simulink model "AF_Sim_March_27"  (R2019b)
settings: Solver=VariableStepAuto  StartTime=0.0  StopTime=200  RelTol=1e-3
values from neighbouring files (symbols this model uses):
  u0 = [ 1.29  -0.1174  0  0]    [AF_Sim_Init.m]    (also in EOM.m = [1.29, -0.1174, 0, 0, -0.0153]; LiftDragMoment.m = [P Q R V beta alpha mu gamma chi zeta eta h]; testrun.m = [1.29, -0.1174, 0,  0, 64.828,     0,  -0.0153, 0,  0,  0,  )
  uin = [0, 0, 0, 0]    [AF_Sim_Init.m]    (also in LiftDragMoment.m = [d_th d_e d_r d_a]; testrun.m = zeros(1,16))
libraries: simulink x1
settings Model: Creator=hyeokjae  LastModifiedBy=chris
settings DebuggingCC: UnderSpecifiedDimensionMsg=warning
settings SFSimCC: CustomCodeUndefinedFunction=UseInterfaceOnly

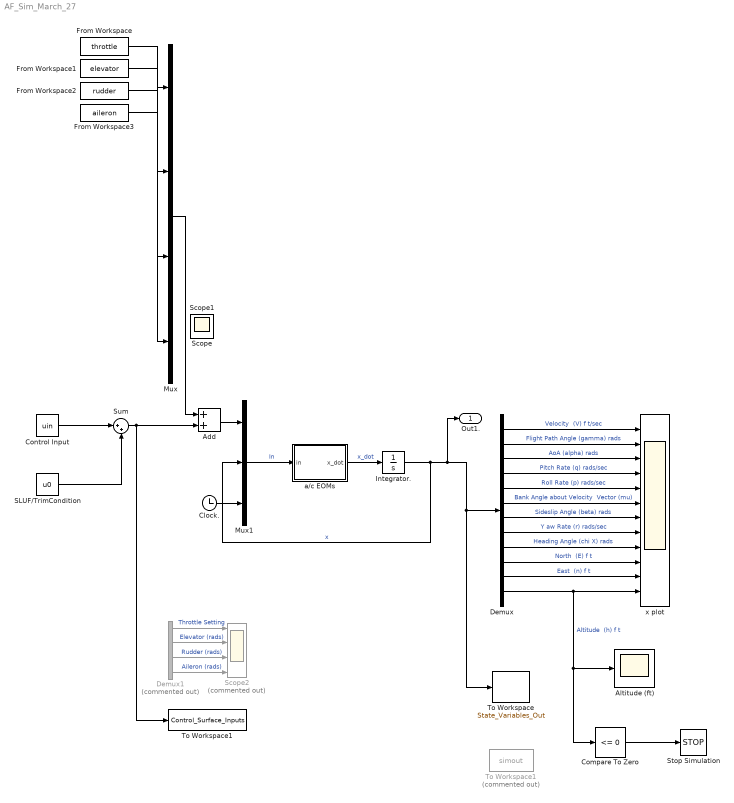
== system AF_Sim_March_27 ==
  Add : Sum
  Altitude (ft) : Scope
  Clock. : Clock
      settings: Decimation=100
  "Compare To Zero " : simulink/Logic and Bit Operations/Compare To Zero  relop=<=  OutDataTypeStr=boolean
  Control Input : Constant  Value=uin
  Demux : Demux  Outputs=12
  Demux1 : Demux  Commented=on
  From Workspace : FromWorkspace  VariableName=throttle  SampleTime=300
  From Workspace1 : FromWorkspace  VariableName=elevator  SampleTime=300
  From Workspace2 : FromWorkspace  VariableName=rudder  SampleTime=300
  From Workspace3 : FromWorkspace  VariableName=aileron  SampleTime=300
  Integrator. : Integrator
  Mux : Mux
  Mux1 : Mux  Inputs=3
  "SLUF/TrimCondition " : Constant  Value=u0
  Scope2 : Scope  Commented=on  NumInputPorts=4
  "Stop Simulation " : Stop
  Sum : Sum  Inputs=|++
  "To Workspace " : ToWorkspace  VariableName=State_Variables_Out  SampleTime=-1
      settings: Save2DSignal=2-D array (concatenate along first dimension)
  To Workspace1 : ToWorkspace  Commented=on  VariableName=simout  SaveFormat=Timeseries  SampleTime=-1
  "To Workspace1 " : ToWorkspace  VariableName=Control_Surface_Inputs  SampleTime=-1
      settings: Save2DSignal=2-D array (concatenate along first dimension)
  a/c EOMs : MATLAB Function  TreatAsAtomicUnit=on
  x plot : Scope  NumInputPorts=12
  Out1. : Outport  VectorParamsAs1DForOutWhenUnconnected=off
  Scope : Scope
  Scope1 : Scope
  wires:
  Control Input/1 -> Sum/1
  "SLUF/TrimCondition "/1 -> Sum/2
  Sum/1 -> "To Workspace1 "/1, Add/2
  Mux1/1 -> a/c EOMs/1(in)  "In"
  a/c EOMs/1(x_dot) -> Integrator./1  "x_dot"
  Integrator./1 -> Mux1/2, Out1./1, "To Workspace "/1, Demux/1  "x"
  Demux/1 -> x plot/1  "Velocity  (V) f t/sec"
  Demux/2 -> x plot/2  "Flight Path Angle (gamma) rads"
  Demux/3 -> x plot/3  "AoA (alpha) rads"
  Demux/4 -> x plot/4  "Pitch Rate (q) rads/sec"
  Demux/5 -> x plot/5  "Roll Rate (p) rads/sec"
  Demux/6 -> x plot/6  "Bank Angle about Velocity  Vector (mu)"
  Demux/7 -> x plot/7  "Sideslip Angle (beta) rads"
  Demux/8 -> x plot/8  "Y aw Rate (r) rads/sec"
  Demux/9 -> x plot/9  "Heading Angle (chi X) rads"
  Demux/10 -> x plot/10  "North  (E) f t"
  Demux/11 -> x plot/11  "East  (n) f t"
  Demux/12 -> "Compare To Zero "/1, Altitude (ft)/1, x plot/12  "Altitude  (h) f t"
  Clock./1 -> Mux1/3
  "Compare To Zero "/1 -> "Stop Simulation "/1
  Demux1/1 -> Scope2/1  "Throttle Setting"
  Demux1/2 -> Scope2/2  "Elevator (rads)"
  Demux1/3 -> Scope2/3  "Rudder (rads)"
  Demux1/4 -> Scope2/4  "Aileron (rads)"
  Add/1 -> Mux1/1
  Mux/1 -> Add/1
  From Workspace/1 -> Mux/1
  From Workspace3/1 -> Mux/4
  From Workspace2/1 -> Mux/3
  From Workspace1/1 -> Mux/2

== matlab function AF_Sim_March_27/a//c EOMs ==
  data: in input; x_dot output
function x_dot = fcn(in)

%AERE 531 Modified Sweep Angle Group
%This function takes inputs in the form of trim conditions (throttle, rudder, elevator...
%and aileron) and control input and outputs flight derivatives for use
%in the simulink model

%The equations used below are grouped together (17-25) and (26-33) as referrenced
%in "Development of Small Unmanned Aerial Vehicle Research Platform:
%Modeling and Simulating with Flight Test Validation"

%global manuever alpha_dot;
x_dot = zeros(12,1);

alpha_dot = 0;

%temporary input vector
%u0 = [1.29, -0.1174, 0,  0, 64.828,     0,  -0.0153, 0,  0,  0,     0, 0,   0,     0,    0, 1119, 100];
    % [T,     de,    dr, da, V,      gamma,  AoA,     q,  p, mu,  beta, r, chi, north, east,    h, clock-input]
   

   
%in = u0;


% PARSING INPUTS
%=============================================================
T   = in(1); %Thrust
de  = in(2); %Elevator deflection (down is +) {deg}
drt = in(3); %Rudder deflection {deg}
da  = in(4); %Aileron deflection {deg}

V       = in(5);  %Velocity {ft/s}
gamma   = in(6);  %Flight path angle {rad}
alpha   = in(7);  %Angle of attack {rad}
q       = in(8);  %Pitch Rate {rad/s}
p       = in(9);  %Roll Rate {rad/s}
mu      = in(10); %Bank Angle (About Velocity Vector) {rad}
beta    = in(11); %Sideslip Angle {rad}
r       = in(12); %Yaw Rate {rad/s}
chi     = in(13); %Heading angle {rads}
north   = in(14); %North Position {ft}
east    = in(15); %East Position {ft}
h       = in(16); %Altitude {ft}

tm = in(17);

% ATMOSPHERIC PROPERTIES
%=============================================================
rho = 0.0023081;    %Air Density (slugs per ft^3) -> do we want to make this a function of height?
g = 32.17;          %ft/s^2


% AIRCRAFT PROPERTIES
%==============================================================


m = 0.487669;       %Slugs - empty mass w/o fuel
Iyy = 1.5523;       %Inertia found with empty mass
Ixx = 1.948;        %Inertia
Izz = 1.9166;       %Inertia
Ixz = 0;            %Assumed zero due to symmetric aircraft

S = 10.56;          %Wing area - square feet
b = 9.16;           % Wing span - feet


CLow = 0.421;       %Wing coefficient of lift at 0deg AoA
CLaw = 4.59;        %Wing coefficient of lift per AoA
CDminw = 0.011;     %wing minimum coefficient of drag
ARw = (b^2)/S;      %Wing aspect ratio
e = 0.75;           %Span efficiency - ESTIMATION
Kw = 1/(pi*ARw*e);  %
Cmw = -0.005;       %Wing moment coefficient
cgw = -(5/12);      %Distance aero center is back from cg - 5 inches
c = (16/12);        %Root chord of wing (16") - feet
lambda = 0.72955;   %Taper ratio from S = (Cr*(1+lambda)*b)/2
CLat = 0.76;        %Vert tail coefficient of lift per AoA
CDmint = 0.002;     %vert tail minimum coeffcient of drag
Kt = 0.446;         %TO DO - MORE CALC?
it = deg2rad(2);    %Tail incidence 2 degrees to radians
Te = 0.422;         %Tail control surface effectiveness (??)
nt = 1;             %??
St = S;             %Horizontal tail area square feet = ref area (??)
cgt = 3.5;          %Distance tail aero center back from a/c cg

CLavt = 0.0969;     %Vertical tail coefficient of lift per AoA(??)
CDminvt = 0.001;    %vert tail min coefficient of drag (??)
Svt = S;            %Ref area of vertical tail = ref area (??)
Tr = 0.434;         %Name??
nvt = nt;           %same as hori tail (??)
cgvt = cgt;         %same as hori tail (??)

Cmaf = 0.114;       %fuselage moment coefficient
CDf = 0.005;        %Fuselage coefficient of drag

Cnda = -0.0128;     %per rad (??)
Clda = 0.244;       %per rad (??)


%Eqns 17-25
%Calculating necessary coefficients for use in Lift, Drag, and Moment
%equations
CLw=CLow+CLaw*alpha; %Coefficient of lift due to wing
CDw=CDminw+Kw*CLw^2; %Coefficient of drag due to wing
E=2*(CLow+CLaw*(alpha-alpha_dot*(cgt+cgw)/V))/(pi*ARw); %Not sure what to call this variable
alphat=alpha+it+Te*de+q*cgt/V-E; %angle of attack at horizontal tail
CLt=CLat*alphat; %Coefficient of lift due to horizonatl tail
CDt=CDmint+Kt*CLt^2; %Coefficient of drag due to horizontal tail
Cmf=Cmaf*alpha; %Moment coefficient due to fueselage 
CDvt=CDminvt; %Coefficient of drag due to vertical tail
Clp=-1/12*CLaw*(1+3*lambda)/(1+lambda); 

Clb=-.1; %rolling moment coefficient due to sideslip beta
Clr=.01;

%Eqns 26 - 33
%Forces and moments due to wing, horizontal and vertical tail, and
%fuselage:
qb=.5*rho*V^2; %q bar (dynamic pressure)
Lw=qb*S*CLw;   %lift due to wing
Dw=qb*S*CDw;   %drag due to wing
Mw=qb*S*c*Cmw; %pitching moment due to wing
Lt=nt*qb*St*CLt; %lift due to horizontal tail
Dt=nt*qb*St*CDt; %drag due to horizontal tai
Df=qb*S*CDf;    %drag due to fuselage
Mf=qb*S*c*Cmf;  %moment due to fuselage
Dvt=nt*qb*Svt*CDvt; %drag due to vertical tail

% Calculate Forces and Moments
% Total Lift
L=Lw+Lt*cos(E-q*cgt/V)-(Dt+Dvt)*sin(E-q*cgt/V);
% Total Drag
D=Dw+(Dt+Dvt)*cos(E-q*cgt/V)+Lt*sin(E-q*cgt/V)+Df;
% Total Side Force
Y=nvt*qb*Svt*CLavt*(-beta+Tr*drt+r*cgvt/V);
% Total Pitching Moment
Mc=Lw*cgw*cos(alpha)+Dw*cgw*sin(alpha)+Mw-Lt*cgt*cos(alpha-E+q*cgt/V)-(Dt+Dvt)*cgt*sin(alpha-E+q*cgt/V)+Mf;
% Total Yaw Moment
Nc=-qb*nvt*Svt*CLavt*(-beta+Tr*drt+r*cgvt/V)*cgvt+(-qb*S*b*Cnda*da);
% Total Roll Moment
Lc=qb*S*b^2/(2*V)*(Clp*p+2*V/b*Clb*beta+Clr*drt+Clda*da*2*V/b);




% -=-=-=-=-=- NONLINEAR 6-DOF EQUATION OF MOTION (EOMs) -=-=-=-=-=-=-=-=-
%
% These are the state derivative equations; the comment names the state,
% but the equation is for its derivative (rate)
%
% The equations are arranged by aircraft mode
%
% NOTE: These assume that Ixz=0, if not, then eq's need to be modified
% Longitudinal (phugoid and short period): V, gamma, q, alpha
% Phugoid: V, gamma
 % Velocity
 V_dot=1/m*(-D*cos(beta)+Y*sin(beta)+T*cos(beta)*cos(alpha))-...
 g*sin(gamma);
 % Flight Path Angle
 gamma_dot=1/(m*V)*(-D*sin(beta)*sin(mu)-Y*sin(mu)*cos(beta)...
 +L*cos(mu)+T*(cos(mu)*sin(alpha)+sin(mu)*sin(beta)*cos(alpha)))...
 -g/V*cos(gamma);
% Short Period: alpha, q
 % Angle of Attach
 alpha_dot=q-tan(beta)*(p*cos(alpha)+r*sin(alpha))-1/(m*V*cos(beta))...
 *(L+T*sin(alpha))+g*cos(gamma)*cos(mu)/(V*cos(beta));
 % Pitch Rate
 q_dot=Mc/Iyy+1/Iyy*(Izz*p*r-Ixx*r*p);
% Lateral (roll) - Directional (yaw): p, mu, beta, r
% Roll: p, mu
 % Roll Rate
 p_dot=Lc/Ixx+1/Ixx*(Iyy*r*q-Izz*q*r);

 % Bank Angle (about velocity vector)
 mu_dot=1/cos(beta)*(p*cos(alpha)+r*sin(alpha))+1/(m*V)*(D*sin(beta)...
 *cos(mu)*tan(gamma)+Y*tan(gamma)*cos(mu)*cos(beta)+L*(tan(beta)+...
 tan(gamma)*sin(mu))+T*(sin(alpha)*tan(gamma)*sin(mu)+sin(alpha)*...
 tan(beta)-cos(alpha)*tan(gamma)*cos(mu)*sin(beta)))-...
 g/V*cos(gamma)*cos(mu)*tan(beta);

% Dutch Roll: beta, r
 % Side Slip Angle
 beta_dot=-r*cos(alpha)+p*sin(alpha)+1/(m*V)*(D*sin(beta)+Y*cos...
 (beta)-T*sin(beta)*cos(alpha))+g/V*cos(gamma)*sin(mu);

 % Yaw Rate

 r_dot=Nc/Izz+1/Izz*(Ixx*p*q-Iyy*p*q);

% Heading Angle (from North)
 chi_dot=1/(m*V*cos(gamma))*(D*sin(beta)*cos(mu)+Y*cos(mu)*cos(beta)...
 +L*sin(mu)+T*(sin(mu)*sin(alpha)-cos(mu)*sin(beta)*cos(alpha)));

% Kinematic Equations
 % North Position
 n_dot=V*cos(gamma)*cos(chi);

 % East Position
 e_dot=V*cos(gamma)*sin(chi);

 % Altitude
 h_dot=V*sin(gamma);

% Pack derivatives into output vector x_dot
 x_dot(1) = V_dot;
 x_dot(2) = gamma_dot;
 x_dot(3) = alpha_dot;
 x_dot(4) = q_dot;
 x_dot(5) = p_dot;
 x_dot(6) = mu_dot;
 x_dot(7) = beta_dot;
 x_dot(8) = r_dot;
 x_dot(9) = chi_dot;
 x_dot(10) = n_dot;
 x_dot(11) = e_dot;
 x_dot(12) = h_dot;
 
end
